simulink model "sim1"  (R2024a)
settings: Solver=FixedStepAuto  StartTime=0.0  StopTime=100000.0  FixedStep=1e-3  RelTol=1e-3
InitFcn:
  | % a0=9; % (1),(2)
  | a0=-9; % (3)
  | % a1=6; % (1),(2)
  | a1=-6; % (3)
  | b0=9;
  | bmin=1;
  | km1=6;
  | km0=9;
  | k0=1;
settings Model: Creator=alexe  LastModifiedBy=alexe

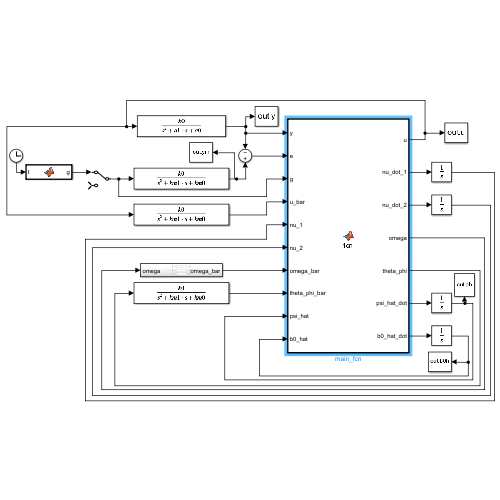
[thumbnail: Simulink's stored preview of the top-level diagram]
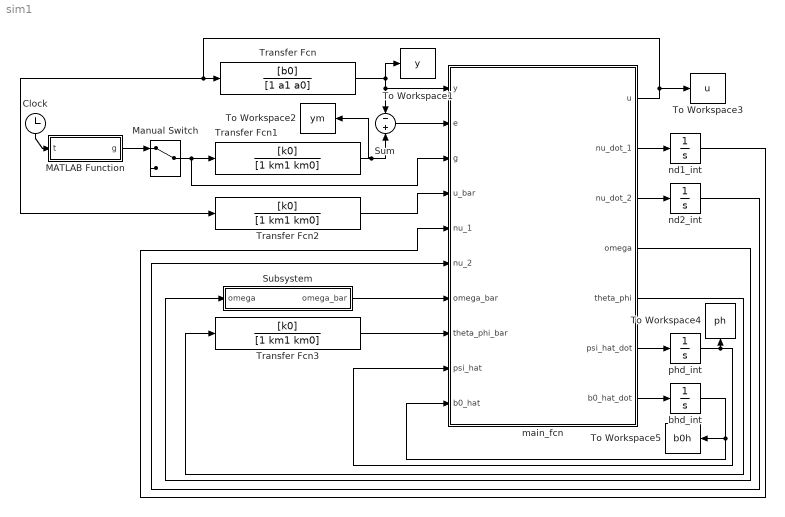
== system sim1 ==
  Clock : Clock
  MATLAB Function : MATLAB Function  TreatAsAtomicUnit=on
  Manual Switch : ManualSwitch
  Subsystem : Subsystem
  Sum : Sum  Inputs=-+
  To Workspace1 : ToWorkspace  VariableName=y  SaveFormat=Structure With Time  SampleTime=-1
  To Workspace2 : ToWorkspace  VariableName=ym  SaveFormat=Structure With Time  SampleTime=-1
  To Workspace3 : ToWorkspace  VariableName=u  SaveFormat=Structure With Time  SampleTime=-1
  To Workspace4 : ToWorkspace  VariableName=ph  SaveFormat=Structure With Time  SampleTime=-1
  To Workspace5 : ToWorkspace  VariableName=b0h  SaveFormat=Structure With Time  SampleTime=-1
  Transfer Fcn : TransferFcn  Numerator=[b0]  Denominator=[1 a1 a0]
  Transfer Fcn1 : TransferFcn  Numerator=[k0]  Denominator=[1 km1 km0]
  Transfer Fcn2 : TransferFcn  Numerator=[k0]  Denominator=[1 km1 km0]
  Transfer Fcn3 : TransferFcn  Numerator=[k0]  Denominator=[1 km1 km0]
  bhd_int : Integrator  InitialCondition=10
  main_fcn : MATLAB Function  TreatAsAtomicUnit=on
  nd1_int : Integrator
  nd2_int : Integrator
  phd_int : Integrator  InitialCondition=[0;0;0]
  wires:
  Clock/1 -> MATLAB Function/1(t)
  Transfer Fcn/1 -> To Workspace1/1, Sum/1, main_fcn/1(y)
  Transfer Fcn1/1 -> To Workspace2/1, Sum/2
  Manual Switch/1 -> main_fcn/3(g), Transfer Fcn1/1
  MATLAB Function/1(g) -> Manual Switch/1
  Sum/1 -> main_fcn/2(e)
  Transfer Fcn2/1 -> main_fcn/4(u_bar)
  main_fcn/1(u) -> To Workspace3/1, Transfer Fcn2/1, Transfer Fcn/1
  main_fcn/2(nu_dot_1) -> nd1_int/1
  main_fcn/3(nu_dot_2) -> nd2_int/1
  main_fcn/6(psi_hat_dot) -> phd_int/1
  main_fcn/7(b0_hat_dot) -> bhd_int/1
  bhd_int/1 -> To Workspace5/1, main_fcn/10(b0_hat)
  phd_int/1 -> To Workspace4/1, main_fcn/9(psi_hat)
  Transfer Fcn3/1 -> main_fcn/8(theta_phi_bar)
  main_fcn/5(theta_phi) -> Transfer Fcn3/1
  nd2_int/1 -> main_fcn/6(nu_2)
  nd1_int/1 -> main_fcn/5(nu_1)
  main_fcn/4(omega) -> Subsystem/1(omega)
  Subsystem/1(omega_bar) -> main_fcn/7(omega_bar)

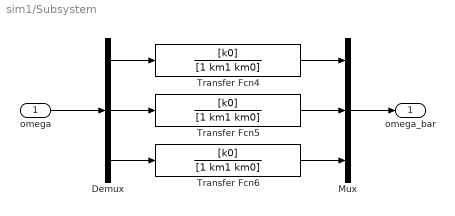
== system sim1/Subsystem ==
  omega : Inport
  Demux : Demux  Outputs=3
  Mux : Mux  Inputs=3
  Transfer Fcn4 : TransferFcn  Numerator=[k0]  Denominator=[1 km1 km0]
  Transfer Fcn5 : TransferFcn  Numerator=[k0]  Denominator=[1 km1 km0]
  Transfer Fcn6 : TransferFcn  Numerator=[k0]  Denominator=[1 km1 km0]
  omega_bar : Outport
  wires:
  Demux/1 -> Transfer Fcn4/1
  Transfer Fcn6/1 -> Mux/3
  Mux/1 -> omega_bar/1
  Transfer Fcn4/1 -> Mux/1
  Demux/3 -> Transfer Fcn6/1
  Demux/2 -> Transfer Fcn5/1
  omega/1 -> Demux/1
  Transfer Fcn5/1 -> Mux/2

== matlab function sim1/MATLAB Function ==
  data: t input; g output
function g = set_signal(t)

g = 0.4*sin(3*t)+cos(0.1*t);

== matlab function sim1/main_fcn ==
  data: y input; e input; g input; u_bar input; u output; nu_1 input; nu_2 input; omega_bar input; theta_phi_bar input; psi_hat input; nu_dot_1 output; nu_dot_2 output; omega output; theta_phi output; psi_hat_dot output; b0_hat input; b0_hat_dot output; k0 parameter; bmin parameter
function [u,nu_dot_1,nu_dot_2,omega,theta_phi, ...
    psi_hat_dot,b0_hat_dot] = fcn(y,e,g,u_bar, ...
    nu_1, nu_2,omega_bar,theta_phi_bar,...
    psi_hat,b0_hat,k0, bmin)
Lambda = -k0;
omega = [nu_1', nu_2', y]';

u = (-psi_hat'*omega + k0*g)/b0_hat;

nu_dot_1 = Lambda*nu_1 + u;
nu_dot_2 = Lambda*nu_2 + y;

theta_hat = [psi_hat; b0_hat];
omega_bar_p = [-omega_bar; -u_bar];

omega_p = [-omega; -u];

theta_phi = theta_hat'*omega_p;

e_hat = e - theta_hat'*omega_bar_p + theta_phi_bar;

gamma1 = 1000;
gamma2 = 1;

psi_hat_dot = -gamma1*omega_bar / ...
    (1 + omega_bar'*omega_bar)*e_hat;
b0_hat_dot = 10;

if b0_hat >= bmin
    b0_hat_dot = -gamma2*u_bar / ...
        (1 + omega_bar'*omega_bar)*e_hat;
elseif b0_hat<bmin
    b0_hat_dot=0;
end
